simulink model "v_1_VTOL_PLANT_DDPG_Simulink"  (Simulink 10.3)
settings: Solver=ode45  StartTime=0.0  StopTime=Tf  RelTol=1e-3
values from neighbouring files (symbols this model uses):
  Gain = 1    [DDPG_find_metrics.m]
  pitch0 = 0    [DDPG_find_metrics.m]
libraries: rllib x1
settings Model: Creator=soyde  LastModifiedBy=mluser  MultithreadedSim=on
settings DataIOCC: SaveFormat=Dataset  SignalLoggingSaveFormat=Dataset  ReturnWorkspaceOutputs=on
settings OptimizationCC: ExpressionDepthLimit=128  LifeSpan=auto
settings DebuggingCC: UnderspecifiedInitializationDetection=Simplified  MergeDetectMultiDrivingBlocksExec=error  FcnCallInpInsideContextMsg=error  StateNameClashWarn=none  SFUnexpectedBacktrackingDiag=error  SFNoUnconditionalDefaultTransitionDiag=error  SFExecutionAtInitializationDiag=warning  ArithmeticOperatorsInVariantConditions=error
settings HardwareCC: ProdBitPerPointer=64  ProdBitPerSizeT=64  ProdBitPerPtrDiffT=64  ProdLargestAtomicFloat=Float  ProdIntDivRoundTo=Zero  ProdEndianess=LittleEndian  ProdWordSize=64  ProdHWDeviceType=Intel->x86-64 (Windows64)
settings ModelReferenceCC: PropagateSignalLabelsOutOfModel=on
settings SFSimCC: SimUseLocalCustomCode=on  CustomCodeUndefinedFunction=FilterOut
settings RTWCC: RTWUseLocalCustomCode=on
settings CodeAppCC: StateflowObjectComments=off
settings GRTTargetCC: TargetLangStandard=C99 (ISO)  CombineOutputUpdateFcns=on  GRTInterface=off
settings ConfigComp: CovMetricSettings=dwe  CovSaveCumulativeToWorkspaceVar=off  CovSaveSingleToWorkspaceVar=off  CovExternalEMLEnable=on

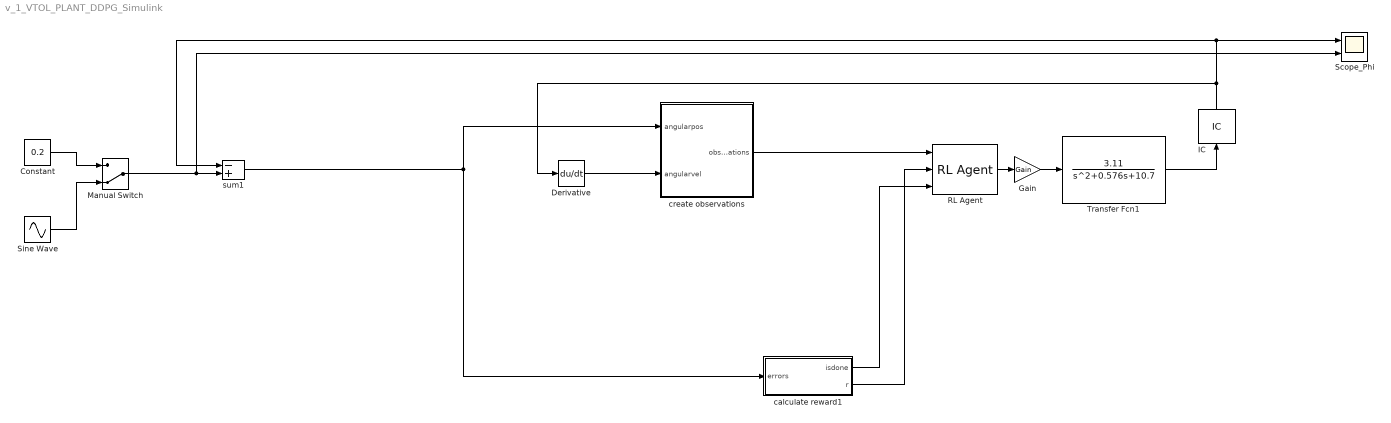
== system v_1_VTOL_PLANT_DDPG_Simulink ==
  Constant : Constant  Value=0.2  SampleTime=0
  Derivative : Derivative
  Gain : Gain  Gain=Gain
  IC : InitialCondition  Value=pitch0
  Manual Switch : ManualSwitch  CurrentSetting=0
  RL Agent : rllib/RL Agent  Agent=saved_agent  ExternalActionAsInput=off  ProvideCumRwd=off  TreatAsDirectFeedthrough=on
  Scope_Phi : Scope  NumInputPorts=2
  Sine Wave : Sin  Amplitude=0.2  Frequency=pi  SampleTime=0
  Transfer Fcn1 : TransferFcn  Numerator=[3.11]  Denominator=[1 0.576 10.7]
  calculate reward1 : Subsystem
  create observations : Subsystem  Variant=on  VariantControlMode=label  VariantControl=Variant1  LabelModeActiveChoice=theta  mask{ThetaObservationHandling=theta}
      mask prompts: ThetaObservationHandling "Select how theta is treated in the observation vector"
      mask init:
      | simulationStatus = get_param(bdroot,'SimulationStatus');
      | 
      | % The active variant can only be modified at edit-time or very early during
      | % the simulink compile stage. 
      | 
      | choice = get_param(gcb,'ThetaObservationHandling');
      | oldVariant = get_param(gcb,'OverrideUsingVariant');
      | 
      | switch choice
      |     case 'theta'
      |     case 'sincos'
      |     otherwise
      |         error('%s is not supported',choice)
      | end
      | set_param(gcb,'OverrideUsingVariant',choice);
      mask TypeOptions ThetaObservationHandling: theta | sincos
  sum1 : Sum  Inputs=-+
  wires:
  Manual Switch/1 -> Scope_Phi/2, sum1/2
  sum1/1 -> calculate reward1/1(errors), create observations/1("angularpos ")
  create observations/1(" observations") -> RL Agent/1
  calculate reward1/1(isdone) -> RL Agent/3
  calculate reward1/2(r) -> RL Agent/2
  Transfer Fcn1/1 -> IC/1
  IC/1 -> sum1/1, Scope_Phi/1, Derivative/1
  RL Agent/1 -> Gain/1
  Derivative/1 -> create observations/2("angularvel ")
  Constant/1 -> Manual Switch/1
  Sine Wave/1 -> Manual Switch/2
  Gain/1 -> Transfer Fcn1/1

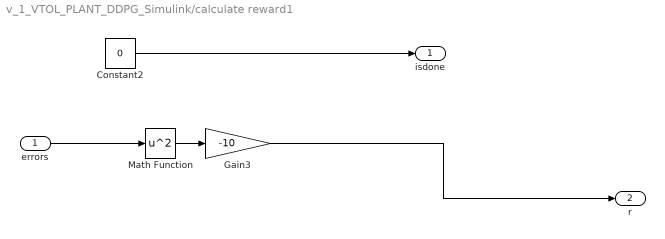
== system v_1_VTOL_PLANT_DDPG_Simulink/calculate reward1 ==
  errors : Inport
  Constant2 : Constant  Value=0
  Gain3 : Gain  Gain=-10
  Math Function : Math  Operator=square  SignedPower=on  SaturateOnIntegerOverflow=on
  isdone : Outport  VectorParamsAs1DForOutWhenUnconnected=off
  r : Outport  Port=2  VectorParamsAs1DForOutWhenUnconnected=off
  wires:
  Constant2/1 -> isdone/1
  errors/1 -> Math Function/1
  Math Function/1 -> Gain3/1
  Gain3/1 -> r/1

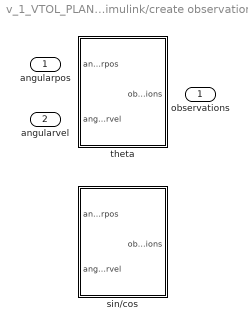
== system v_1_VTOL_PLANT_DDPG_Simulink/create observations ==
  "angularpos " : Inport
  "angularvel " : Inport  Port=2
  sin/cos : Subsystem  VariantControl=sincos
  theta : Subsystem  VariantControl=theta
  " observations" : Outport  VectorParamsAs1DForOutWhenUnconnected=off

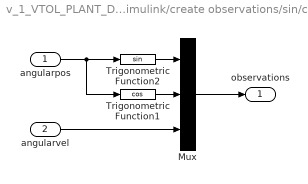
== system v_1_VTOL_PLANT_DDPG_Simulink/create observations/sin/cos ==
  "angularpos " : Inport
  "angularvel " : Inport  Port=2
  Mux : Mux  Inputs=3
  Trigonometric Function1 : Trigonometry  Operator=cos
  Trigonometric Function2 : Trigonometry
  observations : Outport  VectorParamsAs1DForOutWhenUnconnected=off
  wires:
  "angularpos "/1 -> Trigonometric Function1/1, Trigonometric Function2/1
  Mux/1 -> observations/1
  "angularvel "/1 -> Mux/3
  Trigonometric Function2/1 -> Mux/1
  Trigonometric Function1/1 -> Mux/2

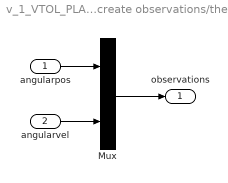
== system v_1_VTOL_PLANT_DDPG_Simulink/create observations/theta ==
  "angularpos " : Inport
  "angularvel " : Inport  Port=2
  Mux : Mux  Inputs=2
  observations : Outport  VectorParamsAs1DForOutWhenUnconnected=off
  wires:
  "angularvel "/1 -> Mux/2
  Mux/1 -> observations/1
  "angularpos "/1 -> Mux/1
